simulink library "NCS_Library"  (R2019a)
settings: Solver=VariableStepAuto  StartTime=0.0  StopTime=10.0  RelTol=1e-3
values from neighbouring files (symbols this model uses):
  A = 10    [Parameter.m]
  band = 100000000    [Parameter.m]
  BER = 0    [Parameter.m]
  c = 5000000    [Parameter.m]
  c1 = 4.33    [Parameter.m]
  c2 = 3.16    [Parameter.m]
  CAN2EthernetDelay = 0.000    (= 0)    [Parameter.m]
  cR = 1.5*10^-3    (= 0.0015)    [Parameter.m]
  cw = (cwE * 2 + cwM * (nW_ges-2))/nW_ges    (= 0.1475)    [Parameter.m]
  cwE = 0.35    [Parameter.m]
  cwM = 0.08    [Parameter.m]
  Cycle_Controller = 0    [Parameter.m]
  CyclePLC = 24/1000    (= 0.024)    [Parameter.m]
  d = 800000    [Parameter.m]
  Dr = 0.92    [Parameter.m]
  Ethernet2CANDelay = 0.005    [Parameter.m]
  F_konst = 70892    [Parameter.m]
  FA = 100000    [Parameter.m]
  FB_WB_max = 10000    [Parameter.m]
  FBel_an = iG*nG*F_KZmax*nBan*R_mR/(Dr/2)    (= 28197.4297239)    [Parameter.m]
  FBel_frei = iG*nG*F_KZmax*nBfrei*R_mW/(Dr/2)    (= 29270.6882948)    [Parameter.m]
  Fmaxdyn = 300000    [Parameter.m]
  g = 9.81    [Parameter.m]
  i = 0    [Parameter.m]
  J = 1/2*mA*(Dr/2)^2    (= 158.7)    [Parameter.m]
  k1 = 0.095    [Parameter.m]
  k2 = 9.26/3.6    (= 2.57222222222)    [Parameter.m]
  k3 = 4.63/3.6    (= 1.28611111111)    [Parameter.m]
  mges = 58000    [Parameter.m]
  mu = [mu1 mu2]    [Parameter.m]
  muBel1 = 0.42    [Parameter.m]
  muBel2 = 0.36    [Parameter.m]
  n = 0.001    [Parameter.m]
  n_Mg = 4    [Parameter.m]
  n_WB = 4    [Parameter.m]
  nA = 4    [Parameter.m]
  nBan = 2    [Parameter.m]
  nBfrei = 3    [Parameter.m]
  nM = 4    [Parameter.m]
  nW_an = 4    [Parameter.m]
  P_max = 8200000    [Parameter.m]
  Q = 10    [Parameter.m]
  r_reib = 600    [Parameter.m]
  rho = 1.08    [Parameter.m]
  rhoL = 1.225    [Parameter.m]
  Size = 8    [Parameter.m]
  slip = [s1 s2]    [Parameter.m]
  tol = 0.05    [Parameter.m]
  v00 = 100/3.6    (= 27.7777777778)    [Parameter.m]
  v_grenz = 60/3.6    (= 16.6666666667)    [Parameter.m]
  v_opt = 75/3.6    (= 20.8333333333)    [Parameter.m]
  W_opt = 0.5    [Parameter.m]
  WB = 1    [Parameter.m]
  y_opt = sqrt(W_opt)/((1+sqrt(W_opt))^2+W_opt)    [Parameter.m]
undefined symbols (not defined in the file or in its folder): BUSCapacity, CableLength, controlGate, D_dyn, D_mg, EnableBurst, EnableToF, entity, Entity_out, Gate, Gate_4, Gate_5, Gate_ACK, Gate_copy, Gate_RX, getData, gettime, I_dyn, I_mg, m, magnitude, P_dyn, P_mg, ReadAttributes, readdata, ReadData, ReadSize, sigbuilder_block, Timeout, ToB, ToF, v0, v_d, v_soll
libraries: simulink x176, $bdroot x102
(part 5 of 12)

== system NCS_Library/Controller/Cookie/Braking Controller/konstante Fahrt ==
  v : Inport
  Add : Sum  Inputs=|+-
  Constant : Constant  Value=v_d
  Display : Display
  Display1 : Display
  Gain : Gain  Gain=-1
  Mux2 : Mux  Inputs=3
  PID Controller : simulink/Continuous/PID Controller  Controller=PID  Form=Parallel  TimeDomain=Continuous-time  SampleTime=-1  IntegratorMethod=Forward Euler  FilterMethod=Forward Euler  ControllerParametersSource=internal  P=0.05  I=0.025  D=0.001  UseFilter=on  N=100  TunerSelectOption=Transfer Function Based (PID Tuner App)  InitialConditionSource=internal  InitialConditionForIntegrator=0  InitialConditionForFilter=0  DifferentiatorICPrevScaledInput=0  ExternalReset=none  TrackingMode=off  Kt=1  LimitOutput=off  UpperSaturationLimit=inf  LowerSaturationLimit=-inf  LinearizeAsGain=on  AntiWindupMode=none  Kb=1  POutMin=[]  POutMax=[]  IOutMin=[]  IOutMax=[]  DOutMin=[]  DOutMax=[]  NOutMin=[]  NOutMax=[]  SumOutMin=[]  SumOutMax=[]  SaturationOutMin=[]  SaturationOutMax=[]  PParamMin=[]  PParamMax=[]  IParamMin=[]  IParamMax=[]  DParamMin=[]  DParamMax=[]  NParamMin=[]  NParamMax=[]  KbParamMin=[]  KbParamMax=[]  KtParamMin=[]  KtParamMax=[]  KbOutMin=[]  KbOutMax=[]  KtOutMin=[]  KtOutMax=[]  IntegratorOutMin=[]  IntegratorOutMax=[]  FilterOutMin=[]  FilterOutMax=[]  SumI1OutMin=[]  SumI1OutMax=[]  SumI2OutMin=[]  SumI2OutMax=[]  SumI3OutMin=[]  SumI3OutMax=[]  SumI4OutMin=[]  SumI4OutMax=[]  SumDOutMin=[]  SumDOutMax=[]  DifferentiatorOutMin=[]  DifferentiatorOutMax=[]  FilterDiffOutCoefMin=[]  FilterDiffOutCoefMax=[]  ReciprocalOutMin=[]  ReciprocalOutMax=[]  SumDenOutMin=[]  SumDenOutMax=[]  SumNumOutMin=[]  SumNumOutMax=[]  DivideOutMin=[]  DivideOutMax=[]  IntegratorContinuousStateAttributes=''  IntegratorStateMustResolveToSignalObject=off  IntegratorRTWStateStorageClass=Auto  FilterContinuousStateAttributes=''  FilterStateMustResolveToSignalObject=off  FilterRTWStateStorageClass=Auto  ParallelPVariant=InternalParameters  IdealPVariant=Disabled  IVariant=InternalParameters  DVariant=InternalParameters  IntegratorVariant=Continuous  SatVariant=Disabled  AWVariant=Passthrough  PCopyVariant=Disabled  TRVariant=Disabled  FdbkBlocksVariant=Forward  IdealPFdbkVariant=Disabled  SatFdbkVariant=Disabled  DerivativeFilterVariant=ContFilter  NVariant=InternalParameters  NCopyVariant=Disabled  FilterICVariant=InternalICsFilter  IntegratorICVariant=InternalICs  ExternalResetVariant=Disabled  TRSumVariant=Passthrough  SumFdbkVariant=Disabled  SumVariant=Sum_PID
  PID Controller1 : simulink/Continuous/PID Controller  Controller=PID  Form=Parallel  TimeDomain=Continuous-time  SampleTime=-1  IntegratorMethod=Forward Euler  FilterMethod=Forward Euler  ControllerParametersSource=internal  P=10  I=100  D=0  UseFilter=on  N=100  TunerSelectOption=Transfer Function Based (PID Tuner App)  InitialConditionSource=internal  InitialConditionForIntegrator=0  InitialConditionForFilter=0  DifferentiatorICPrevScaledInput=0  ExternalReset=none  TrackingMode=off  Kt=1  LimitOutput=off  UpperSaturationLimit=inf  LowerSaturationLimit=-inf  LinearizeAsGain=on  AntiWindupMode=none  Kb=1  POutMin=[]  POutMax=[]  IOutMin=[]  IOutMax=[]  DOutMin=[]  DOutMax=[]  NOutMin=[]  NOutMax=[]  SumOutMin=[]  SumOutMax=[]  SaturationOutMin=[]  SaturationOutMax=[]  PParamMin=[]  PParamMax=[]  IParamMin=[]  IParamMax=[]  DParamMin=[]  DParamMax=[]  NParamMin=[]  NParamMax=[]  KbParamMin=[]  KbParamMax=[]  KtParamMin=[]  KtParamMax=[]  KbOutMin=[]  KbOutMax=[]  KtOutMin=[]  KtOutMax=[]  IntegratorOutMin=[]  IntegratorOutMax=[]  FilterOutMin=[]  FilterOutMax=[]  SumI1OutMin=[]  SumI1OutMax=[]  SumI2OutMin=[]  SumI2OutMax=[]  SumI3OutMin=[]  SumI3OutMax=[]  SumI4OutMin=[]  SumI4OutMax=[]  SumDOutMin=[]  SumDOutMax=[]  DifferentiatorOutMin=[]  DifferentiatorOutMax=[]  FilterDiffOutCoefMin=[]  FilterDiffOutCoefMax=[]  ReciprocalOutMin=[]  ReciprocalOutMax=[]  SumDenOutMin=[]  SumDenOutMax=[]  SumNumOutMin=[]  SumNumOutMax=[]  DivideOutMin=[]  DivideOutMax=[]  IntegratorContinuousStateAttributes=''  IntegratorStateMustResolveToSignalObject=off  IntegratorRTWStateStorageClass=Auto  FilterContinuousStateAttributes=''  FilterStateMustResolveToSignalObject=off  FilterRTWStateStorageClass=Auto  ParallelPVariant=InternalParameters  IdealPVariant=Disabled  IVariant=InternalParameters  DVariant=InternalParameters  IntegratorVariant=Continuous  SatVariant=Disabled  AWVariant=Passthrough  PCopyVariant=Disabled  TRVariant=Disabled  FdbkBlocksVariant=Forward  IdealPFdbkVariant=Disabled  SatFdbkVariant=Disabled  DerivativeFilterVariant=ContFilter  NVariant=InternalParameters  NCopyVariant=Disabled  FilterICVariant=InternalICsFilter  IntegratorICVariant=InternalICs  ExternalResetVariant=Disabled  TRSumVariant=Passthrough  SumFdbkVariant=Disabled  SumVariant=Sum_PID
  Saturation : Saturate  UpperLimit=1  LowerLimit=-1  ZeroCross=off
  Saturation1 : Saturate  UpperLimit=0.01  LowerLimit=0  ZeroCross=off
  fSt1 : Constant  Value=0
  fSt : Outport
  wires:
  Gain/1 -> Saturation/1, Display1/1
  Add/1 -> PID Controller/1, PID Controller1/1, Display/1  "e"
  v/1 -> Add/2  "y_m"
  Constant/1 -> Add/1  "w"
  fSt1/1 -> Mux2/2  "f_St,pneumatic"
  Mux2/1 -> fSt/1
  PID Controller/1 -> Gain/1  "u"
  PID Controller1/1 -> Saturation1/1  "u"
  Saturation/1 -> Mux2/1  "f_St,dyn"
  Saturation1/1 -> Mux2/3  "f_St,mg"

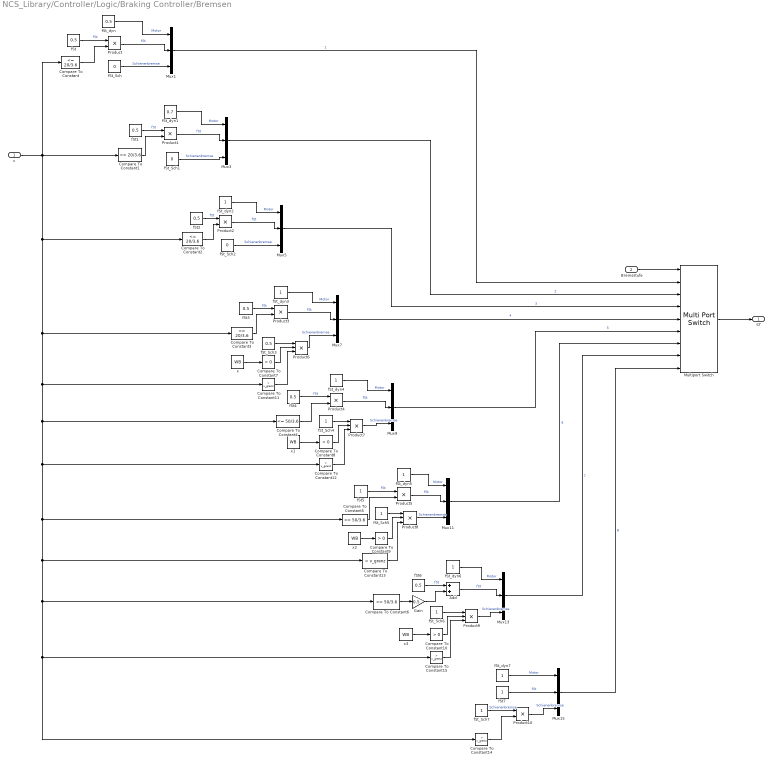
== system NCS_Library/Controller/Logic/Braking Controller/Bremsen ==
  v : Inport
  Bremsstufe : Inport  Port=2
  Add : Sum
  Compare To Constant{,1..3} (4 alike) : simulink/Logic and Bit Operations/Compare To Constant  relop=<=  const=20/3.6  OutDataTypeStr=boolean
  Compare To Constant{7..10} (4 alike) : simulink/Logic and Bit Operations/Compare To Constant  relop=>  const=0  OutDataTypeStr=boolean
  Compare To Constant{11..15} (5 alike) : simulink/Logic and Bit Operations/Compare To Constant  relop=>  const=v_grenz  OutDataTypeStr=boolean
  Compare To Constant4 : simulink/Logic and Bit Operations/Compare To Constant  relop=<=  const=50/3.6  OutDataTypeStr=boolean
  Compare To Constant5 : simulink/Logic and Bit Operations/Compare To Constant  relop=<=  const=50/3.6  OutDataTypeStr=boolean
  Compare To Constant6 : simulink/Logic and Bit Operations/Compare To Constant  relop=<=  const=50/3.6  OutDataTypeStr=boolean
  Gain : Gain  Gain=0.5
  Multiport Switch : MultiPortSwitch  Inputs=8
  Mux{1,3,5,7,9,11,13,15} (8 alike) : Mux  Inputs=3
  Product{,1..5,10} (7 alike) : Product
  Product{6..9} (4 alike) : Product  Inputs=3
  fSt{,1..4,6} (6 alike) : Constant  Value=0.5
  fSt5 : Constant
  fSt7 : Constant
  fSt_Sch : Constant  Value=0
  fSt_Sch1 : Constant  Value=0
  fSt_Sch2 : Constant  Value=0
  fSt_Sch3 : Constant  Value=0.5
  fSt_Sch{4..7} (4 alike) : Constant
  fSt_dyn : Constant  Value=0.5
  fSt_dyn1 : Constant  Value=0.7
  fSt_dyn{2..7} (6 alike) : Constant
  x{,1..3} (4 alike) : Constant  Value=WB
  ST : Outport
  wires:
  Compare To Constant15/1 -> Product9/3
  Compare To Constant14/1 -> Product10/2
  Product10/1 -> Mux15/3  "Schienenbremse"
  Compare To Constant13/1 -> Product8/3
  Compare To Constant12/1 -> Product7/3
  Compare To Constant11/1 -> Product6/3
  Compare To Constant10/1 -> Product9/2
  x3/1 -> Compare To Constant10/1
  fSt_Sch6/1 -> Product9/1
  Compare To Constant9/1 -> Product8/2
  x2/1 -> Compare To Constant9/1
  fSt_Sch5/1 -> Product8/1
  Compare To Constant8/1 -> Product7/2
  x1/1 -> Compare To Constant8/1
  fSt_Sch4/1 -> Product7/1
  Compare To Constant7/1 -> Product6/2
  x/1 -> Compare To Constant7/1
  fSt_Sch3/1 -> Product6/1
  Gain/1 -> Add/2
  fSt6/1 -> Add/1  "fSt"
  Compare To Constant6/1 -> Gain/1
  fSt5/1 -> Product5/1  "fSt"
  Compare To Constant5/1 -> Product5/2
  fSt4/1 -> Product4/1  "fSt"
  Compare To Constant4/1 -> Product4/2
  fSt3/1 -> Product3/1  "fSt"
  Compare To Constant3/1 -> Product3/2
  fSt2/1 -> Product2/1  "fSt"
  Compare To Constant2/1 -> Product2/2
  Compare To Constant1/1 -> Product1/2
  fSt1/1 -> Product1/1  "fSt"
  v/1 -> Compare To Constant1/1, Compare To Constant/1, Compare To Constant2/1, Compare To Constant3/1, Compare To Constant11/1, Compare To Constant4/1, Compare To Constant12/1, Compare To Constant5/1, Compare To Constant14/1, Compare To Constant15/1, Compare To Constant6/1, Compare To Constant13/1
  Compare To Constant/1 -> Product/2
  fSt/1 -> Product/1  "fSt"
  Bremsstufe/1 -> Multiport Switch/1
  Mux15/1 -> Multiport Switch/9  "8"
  fSt_dyn7/1 -> Mux15/1  "Motor"
  fSt_Sch7/1 -> Product10/1  "Schienenbremse"
  fSt7/1 -> Mux15/2  "fSt"
  Mux13/1 -> Multiport Switch/8  "7"
  fSt_dyn6/1 -> Mux13/1  "Motor"
  Product9/1 -> Mux13/3  "Schienenbremse"
  Add/1 -> Mux13/2  "fSt"
  Mux11/1 -> Multiport Switch/7  "6"
  fSt_dyn5/1 -> Mux11/1  "Motor"
  Product8/1 -> Mux11/3  "Schienenbremse"
  Product5/1 -> Mux11/2  "fSt"
  Mux9/1 -> Multiport Switch/6  "5"
  fSt_dyn4/1 -> Mux9/1  "Motor"
  Product7/1 -> Mux9/3  "Schienenbremse"
  Product4/1 -> Mux9/2  "fSt"
  Mux7/1 -> Multiport Switch/5  "4"
  fSt_dyn3/1 -> Mux7/1  "Motor"
  Product6/1 -> Mux7/3  "Schienenbremse"
  Product3/1 -> Mux7/2  "fSt"
  Mux5/1 -> Multiport Switch/4  "3"
  fSt_dyn2/1 -> Mux5/1  "Motor"
  fSt_Sch2/1 -> Mux5/3  "Schienenbremse"
  Product2/1 -> Mux5/2  "fSt"
  Mux3/1 -> Multiport Switch/3  "2"
  fSt_dyn1/1 -> Mux3/1  "Motor"
  fSt_Sch1/1 -> Mux3/3  "Schienenbremse"
  Product1/1 -> Mux3/2  "fSt"
  Mux1/1 -> Multiport Switch/2  "1"
  fSt_dyn/1 -> Mux1/1  "Motor"
  fSt_Sch/1 -> Mux1/3  "Schienenbremse"
  Product/1 -> Mux1/2  "fSt"
  Multiport Switch/1 -> ST/1

== system NCS_Library/Controller/Logic/Braking Controller/Leerlauf ==
  F_B : Constant  Value=0
  Mux1 : Mux  Inputs=3
  fSt : Constant  Value=0
  fSt_Sch : Constant  Value=0
  ST : Outport
  wires:
  Mux1/1 -> ST/1
  fSt_Sch/1 -> Mux1/3  "Schienenbremse"
  fSt/1 -> Mux1/2  "fSt"
  F_B/1 -> Mux1/1  "Motor"

== system NCS_Library/Controller/Logic/Braking Controller/Notbremsung ==
  v : Inport
  Compare To Constant : simulink/Logic and Bit Operations/Compare To Constant  relop=>  const=v_grenz  OutDataTypeStr=boolean
  Mux2 : Mux  Inputs=3
  Product9 : Product
  fSt : Constant
  fSt_Sch : Constant
  fSt_dyn : Constant
  ST : Outport
  wires:
  Compare To Constant/1 -> Product9/2
  v/1 -> Compare To Constant/1
  fSt_Sch/1 -> Product9/1  "Schienenbremse"
  fSt_dyn/1 -> Mux2/1  "fSt_dyn"
  Product9/1 -> Mux2/3  "Schienenbremse"
  fSt/1 -> Mux2/2  "fSt"
  Mux2/1 -> ST/1

== system NCS_Library/Controller/Logic/Braking Controller/konstante Fahrt ==
  v : Inport
  Display{,1..3} (4 alike) : Display
  Fahrwiderstand : Subsystem
  Mux2 : Mux  Inputs=3
  Saturation : Saturate  UpperLimit=1  LowerLimit=0  ZeroCross=off
  Saturation1 : Saturate  UpperLimit=1  LowerLimit=0  ZeroCross=off
  Subsystem : Subsystem
  Subsystem1 : Subsystem
  WB Bremse pro Wagen : Subsystem
  fSt1 : Constant  Value=0
  verfügbare Dynamische Bremskraft : Subsystem
  fSt : Outport
  wires:
  verfügbare Dynamische Bremskraft/1(F_B,dyn_max) -> Subsystem1/2(F_B,dyn_max), Subsystem/2(FB)
  Fahrwiderstand/1(F_W) -> Subsystem1/1(F_W), Subsystem/1(FW)  "FW"
  fSt1/1 -> Mux2/2  "fSt"
  Mux2/1 -> fSt/1
  v/1 -> Subsystem1/4(v), WB Bremse pro Wagen/1(v), Fahrwiderstand/1(v), verfügbare Dynamische Bremskraft/1(v)
  Subsystem/1(Motor) -> Display/1, Saturation/1
  WB Bremse pro Wagen/1(F_B,WB) -> Subsystem1/3(F_B,WB)  "F_B,WB"
  Subsystem1/1(Schienenbremse) -> Display2/1, Saturation1/1
  Saturation/1 -> Display1/1, Mux2/1
  Saturation1/1 -> Display3/1, Mux2/3

== system NCS_Library/Controller/Logic/Subsystem/Triggered Subsystem ==
  In1 : Inport
  Trigger : TriggerPort  VariantControl=Variant
  Out1 : Outport
  wires:
  In1/1 -> Out1/1

== system NCS_Library/Controller/Logic/Subsystem/Triggered Subsystem1 ==
  In1 : Inport
  Trigger : TriggerPort  TriggerType=falling  VariantControl=Variant
  Out1 : Outport
  wires:
  In1/1 -> Out1/1

== system NCS_Library/Controller/Logic/Subsystem1/Triggered Subsystem ==
  In1 : Inport
  Trigger : TriggerPort  VariantControl=Variant
  Out1 : Outport
  wires:
  In1/1 -> Out1/1

== system NCS_Library/Controller/Logic/Subsystem1/Triggered Subsystem1 ==
  In1 : Inport
  Trigger : TriggerPort  TriggerType=falling  VariantControl=Variant
  Out1 : Outport
  wires:
  In1/1 -> Out1/1

== system NCS_Library/Network/Applications/Failure Control/Simulink Function ==
  f : TriggerPort  TriggerType=function-call  IsSimulinkFunction=on  FunctionName=DeleteData  FunctionVisibility=scoped  VariantControl=(inherit)
  Constant : Constant  Value=zeros(3,20)
  y : ArgOut  DisableCoverage=on  PortDimensions=[3 20]  ArgumentName=Data
  wires:
  Constant/1 -> y/1

== system NCS_Library/Network/Applications/Watch Dog/Timeout Watch Dog/GetTime ==
  f : TriggerPort  TriggerType=function-call  VariantControl=(inherit)
      settings: CopyFcn=Stateflow.SLINSF.SimulinkMan.removeBlockPreDeleteFcn  PreDeleteFcn=Stateflow.SLINSF.SimulinkMan.unsafePredeleteFcn
  Digital Clock : DigitalClock  SampleTime=-1
  Time : Outport
  wires:
  Digital Clock/1 -> Time/1

== system NCS_Library/Network/CAN/CAN BUS/Simulink Function ==
  setLossState : TriggerPort  TriggerType=function-call  IsSimulinkFunction=on  FunctionName=setLossState  FunctionVisibility=scoped  VariantControl=Variant
  Constant : Constant
  Constant1 : Constant  Value=0
  Switch : Switch  Criteria=u2 > Threshold  Threshold=LossRate  ZeroCross=off
  Uniform Random Number : UniformRandomNumber  Minimum=0  Seed=724572
  state : ArgOut  ArgumentName=state
  wires:
  Uniform Random Number/1 -> Switch/2
  Constant/1 -> Switch/3
  Constant1/1 -> Switch/1
  Switch/1 -> state/1

== system NCS_Library/Network/CAN/CAN BUS/Simulink Function1 ==
  controlGate : TriggerPort  TriggerType=function-call  IsSimulinkFunction=on  FunctionName=controlGate  FunctionVisibility=scoped  VariantControl=Variant
  Message Send : MessageSend  OutputPortMessageModes=m
      settings: InputPortMap=u1
  u : ArgIn  DisableCoverage=on  ArgumentName=u
  ctrl : Outport
  wires:
  Message Send/1 -> ctrl/1
  u/1 -> Message Send/1

== system NCS_Library/Network/CAN/CAN BUS1/Simulink Function ==
  setLossState : TriggerPort  TriggerType=function-call  IsSimulinkFunction=on  FunctionName=setLossState  FunctionVisibility=scoped  VariantControl=Variant
  Constant : Constant
  Constant1 : Constant  Value=0
  Switch : Switch  Criteria=u2 > Threshold  Threshold=LossRate  ZeroCross=off
  Uniform Random Number : UniformRandomNumber  Minimum=0  Seed=724572
  state : ArgOut  ArgumentName=state
  wires:
  Switch/1 -> state/1
  Constant1/1 -> Switch/1
  Constant/1 -> Switch/3
  Uniform Random Number/1 -> Switch/2

== system NCS_Library/Network/CAN/CAN BUS1/Simulink Function1 ==
  controlGate : TriggerPort  TriggerType=function-call  IsSimulinkFunction=on  FunctionName=controlGate  FunctionVisibility=scoped  VariantControl=Variant
  Message Send : MessageSend  OutputPortMessageModes=m
      settings: InputPortMap=u1
  u : ArgIn  DisableCoverage=on  ArgumentName=u
  ctrl : Outport
  wires:
  u/1 -> Message Send/1
  Message Send/1 -> ctrl/1

== system NCS_Library/Network/CAN/CAN Node 1/Re-Transmission Control ==
  IN : Inport
  ReTX : Inport  Port=2
  Reset : Inport  Port=3
  Discard Saved Message upon Success : EntityGate  InputPortMessageModes=m,m  OutputPortMessageModes=m  OperatingMode=Release gate
  Entity Sink : EntityTerminator  InputPortMessageModes=m  NumberEntitiesArrived=on
      settings: OutputPortMap=o0
  Re-Transmission Decision : EntityOutputSwitch  InputPortMessageModes=m  OutputPortMessageModes=m,m  SwitchAttributeName=Attribute1
  Re-transmit Saved Message upon Failure : EntityGate  InputPortMessageModes=m,m  OutputPortMessageModes=m  OperatingMode=Release gate
  OUT : Outport
  #TX : Outport  Port=2
  wires:
  IN/1 -> Re-Transmission Decision/1
  Re-Transmission Decision/1 -> Re-transmit Saved Message upon Failure/2
  Re-transmit Saved Message upon Failure/1 -> OUT/1
  Re-Transmission Decision/2 -> Discard Saved Message upon Success/2
  Discard Saved Message upon Success/1 -> Entity Sink/1
  Entity Sink/1 -> #TX/1
  ReTX/1 -> Re-transmit Saved Message upon Failure/1
  Reset/1 -> Discard Saved Message upon Success/1

== system NCS_Library/Network/CAN/CAN Node 1/Reception Control/Compute ==
  rx_id : Inport  OutDataTypeStr=double  PortDimensions=1
  loss : Inport  Port=2  OutDataTypeStr=double  PortDimensions=1
  rx_rtr : Inport  Port=3  OutDataTypeStr=double  PortDimensions=1
  rx_data : Inport  Port=4  OutDataTypeStr=double  PortDimensions=1
  tx_id : Inport  Port=5  OutDataTypeStr=double  PortDimensions=1
  tx_rtr : Inport  Port=6  OutDataTypeStr=double  PortDimensions=1
  tx_data : Inport  Port=7  OutDataTypeStr=double  PortDimensions=1
  f : TriggerPort  TriggerType=function-call  VariantControl=Variant
      settings: CopyFcn=Stateflow.SLINSF.SimulinkMan.removeBlockPreDeleteFcn  PreDeleteFcn=Stateflow.SLINSF.SimulinkMan.unsafePredeleteFcn
  Lookup Table : Lookup  InputValues=IDRange  Table=2*ones(1,length(IDRange))-IDSubscription  LUTDesignUseExistingBP=off  LUTDesignAbsError=NaN
  MATLAB Function : MATLAB Function  TreatAsAtomicUnit=on
  Sum : Sum  Inputs=|++
  Status : Outport
  Ack : Outport  Port=2
  wires:
  MATLAB Function/1(ACK) -> Ack/1
  Sum/1 -> Status/1
  tx_rtr/1 -> MATLAB Function/5(RTR1)
  tx_data/1 -> MATLAB Function/6(Data1)
  rx_data/1 -> MATLAB Function/3(Data0)
  loss/1 -> MATLAB Function/7(Loss), Sum/2
  Lookup Table/1 -> Sum/1
  rx_id/1 -> Lookup Table/1, MATLAB Function/1(ID0)
  rx_rtr/1 -> MATLAB Function/2(RTR0)
  tx_id/1 -> MATLAB Function/4(ID1)

== system NCS_Library/Network/CAN/CAN Node 1/Signal To CAN Message ==
  Data : Inport
  Entity Generator : EntityGenerator  OutputPortMessageModes=m  Period=T_Tx  GenerateEntityAtSimulationStart=off  GenerateAction=[entity.ID,entity.RTR,entity.Size,entity.Data,entity.CommDelay,entity.Time, entity.SensorType] = initMessage();  AttributeName=ID|RTR|Size|Data|CommDelay|RndLoss  AttributeInitialValue=1|1|1|1|1|0  EntityType=Bus object  EntityTypeName=CAN_Message  EntityPriority=MsgID
  Set the Attributes of Messages : Subsystem  TreatAsAtomicUnit=on
  MsgOut : Outport
  wires:
  Data/1 -> Set the Attributes of Messages/1(InData)
  Entity Generator/1 -> MsgOut/1

== system NCS_Library/Network/CAN/CAN Node 1/Simulink Function ==
  controlGate : TriggerPort  TriggerType=function-call  IsSimulinkFunction=on  FunctionName=controlGate  FunctionVisibility=scoped  VariantControl=Variant
  Message Send : MessageSend  OutputPortMessageModes=m
      settings: InputPortMap=u1
  u : ArgIn  DisableCoverage=on  ArgumentName=u
  ctrl : Outport
  wires:
  Message Send/1 -> ctrl/1
  u/1 -> Message Send/1

== system NCS_Library/Network/CAN/CAN Node 1/Simulink Function1 ==
  getData : TriggerPort  TriggerType=function-call  IsSimulinkFunction=on  FunctionName=getData  FunctionVisibility=scoped  VariantControl=Variant
  Mux : Mux  Inputs=3
  u : ArgIn  DisableCoverage=on  ArgumentName=u
  u1 : ArgIn  DisableCoverage=on  Port=2  PortDimensions=[3 1]  ArgumentName=f_St
  data : Outport
  f_St : Outport  Port=2
  wires:
  u/1 -> Mux/1, Mux/3, Mux/2
  u1/1 -> f_St/1
  Mux/1 -> data/1

== system NCS_Library/Network/CAN/CAN Node 2/Re-Transmission Control ==
  IN : Inport
  ReTX : Inport  Port=2
  Reset : Inport  Port=3
  Discard Saved Message upon Success : EntityGate  InputPortMessageModes=m,m  OutputPortMessageModes=m  OperatingMode=Release gate
  Entity Sink : EntityTerminator  InputPortMessageModes=m  NumberEntitiesArrived=on
      settings: OutputPortMap=o0
  Re-Transmission Decision : EntityOutputSwitch  InputPortMessageModes=m  OutputPortMessageModes=m,m  SwitchAttributeName=Attribute1
  Re-transmit Saved Message upon Failure : EntityGate  InputPortMessageModes=m,m  OutputPortMessageModes=m  OperatingMode=Release gate
  OUT : Outport
  #TX : Outport  Port=2
  wires:
  Reset/1 -> Discard Saved Message upon Success/1
  ReTX/1 -> Re-transmit Saved Message upon Failure/1
  Entity Sink/1 -> #TX/1
  Discard Saved Message upon Success/1 -> Entity Sink/1
  Re-Transmission Decision/2 -> Discard Saved Message upon Success/2
  Re-transmit Saved Message upon Failure/1 -> OUT/1
  Re-Transmission Decision/1 -> Re-transmit Saved Message upon Failure/2
  IN/1 -> Re-Transmission Decision/1

== system NCS_Library/Network/CAN/CAN Node 2/Reception Control/Compute ==
  rx_id : Inport  OutDataTypeStr=double  PortDimensions=1
  loss : Inport  Port=2  OutDataTypeStr=double  PortDimensions=1
  rx_rtr : Inport  Port=3  OutDataTypeStr=double  PortDimensions=1
  rx_data : Inport  Port=4  OutDataTypeStr=double  PortDimensions=1
  tx_id : Inport  Port=5  OutDataTypeStr=double  PortDimensions=1
  tx_rtr : Inport  Port=6  OutDataTypeStr=double  PortDimensions=1
  tx_data : Inport  Port=7  OutDataTypeStr=double  PortDimensions=1
  f : TriggerPort  TriggerType=function-call  VariantControl=Variant
      settings: CopyFcn=Stateflow.SLINSF.SimulinkMan.removeBlockPreDeleteFcn  PreDeleteFcn=Stateflow.SLINSF.SimulinkMan.unsafePredeleteFcn
  Lookup Table : Lookup  InputValues=IDRange  Table=2*ones(1,length(IDRange))-IDSubscription  LUTDesignUseExistingBP=off  LUTDesignAbsError=NaN
  MATLAB Function : MATLAB Function  TreatAsAtomicUnit=on
  Sum : Sum  Inputs=|++
  Status : Outport
  Ack : Outport  Port=2
  wires:
  tx_id/1 -> MATLAB Function/4(ID1)
  rx_rtr/1 -> MATLAB Function/2(RTR0)
  rx_id/1 -> MATLAB Function/1(ID0), Lookup Table/1
  Lookup Table/1 -> Sum/1
  loss/1 -> Sum/2, MATLAB Function/7(Loss)
  rx_data/1 -> MATLAB Function/3(Data0)
  tx_data/1 -> MATLAB Function/6(Data1)
  tx_rtr/1 -> MATLAB Function/5(RTR1)
  Sum/1 -> Status/1
  MATLAB Function/1(ACK) -> Ack/1

== system NCS_Library/Network/CAN/CAN Node 2/Signal To CAN Message ==
  Data : Inport
  Entity Generator : EntityGenerator  OutputPortMessageModes=m  Period=T_Tx  GenerateEntityAtSimulationStart=off  GenerateAction=[entity.ID,entity.RTR,entity.Size,entity.Data,entity.CommDelay,entity.Time, entity.SensorType] = initMessage();  AttributeName=ID|RTR|Size|Data|CommDelay|RndLoss  AttributeInitialValue=1|1|1|1|1|0  EntityType=Bus object  EntityTypeName=CAN_Message  EntityPriority=MsgID
  Set the Attributes of Messages : Subsystem  TreatAsAtomicUnit=on
  MsgOut : Outport
  wires:
  Entity Generator/1 -> MsgOut/1
  Data/1 -> Set the Attributes of Messages/1(InData)

== system NCS_Library/Network/CAN/CAN Node 2/Simulink Function ==
  controlGate : TriggerPort  TriggerType=function-call  IsSimulinkFunction=on  FunctionName=controlGate  FunctionVisibility=scoped  VariantControl=Variant
  Message Send : MessageSend  OutputPortMessageModes=m
      settings: InputPortMap=u1
  u : ArgIn  DisableCoverage=on  ArgumentName=u
  ctrl : Outport
  wires:
  u/1 -> Message Send/1
  Message Send/1 -> ctrl/1

== system NCS_Library/Network/CAN/CAN Node 2/Simulink Function1 ==
  getData : TriggerPort  TriggerType=function-call  IsSimulinkFunction=on  FunctionName=getData  FunctionVisibility=scoped  VariantControl=Variant
  Mux : Mux  Inputs=3
  u : ArgIn  DisableCoverage=on  ArgumentName=u
  u1 : ArgIn  DisableCoverage=on  Port=2  PortDimensions=[3 1]  ArgumentName=f_St
  data : Outport
  f_St : Outport  Port=2
  wires:
  Mux/1 -> data/1
  u1/1 -> f_St/1
  u/1 -> Mux/2, Mux/3, Mux/1

== system NCS_Library/Network/CAN/CAN Node 3/ACK Takt ==
  In : Inport
  Entity Takt : EntityGenerator  OutputPortMessageModes=m  TimeSource=Signal port  Period=7  AttributeName=entity  EntityTypeName=gate  EntityPriority=10  DataInitialValue=1
      settings: InputPortMap=u1
  Entity Terminator13 : EntityTerminator  InputPortMessageModes=m
  Gate ACK : EntityGate  InputPortMessageModes=m,m  OutputPortMessageModes=m
  Offset [s] : Constant  Value=Offset
  Server ACK : EntityServer  InputPortMessageModes=m  OutputPortMessageModes=m  Capacity=1  ServiceTimeValue=0  EntryAction=Gate_ACK(ideal);
  Server Offset : EntityServer  InputPortMessageModes=n,m  OutputPortMessageModes=m  Capacity=inf  ServiceTimeSource=Signal port  ServiceTimeValue=5
      settings: InputPortMap=u0,u2
  Server Takt : EntityServer  InputPortMessageModes=m  OutputPortMessageModes=m  Capacity=1  ServiceTimeValue=0.001  ServiceTimeAttributeName=CommDelay  EntryAction=Gate_ACK(1);  ExitAction=Gate_ACK(ideal);  SortingAttributeName=ID
  Simulink Function3 : Subsystem  TreatAsAtomicUnit=on
  Takt [s] : Constant  Value=Takt
  Out : Outport
  wires:
  Offset [s]/1 -> Server Offset/1
  Takt [s]/1 -> Entity Takt/1
  Server Takt/1 -> Entity Terminator13/1
  Server Offset/1 -> Server Takt/1
  Entity Takt/1 -> Server Offset/2
  Simulink Function3/1(ctrl) -> Gate ACK/1
  In/1 -> Gate ACK/2
  Gate ACK/1 -> Server ACK/1
  Server ACK/1 -> Out/1

== system NCS_Library/Network/CAN/CAN Node 3/RX Takt ==
  In : Inport
  Entity Takt : EntityGenerator  OutputPortMessageModes=m  TimeSource=Signal port  Period=7  AttributeName=entity  EntityTypeName=gate  EntityPriority=10  DataInitialValue=1
      settings: InputPortMap=u1
  Entity Terminator13 : EntityTerminator  InputPortMessageModes=m
  Gate RX : EntityGate  InputPortMessageModes=m,m  OutputPortMessageModes=m
  Offset [s] : Constant  Value=Offset
  Server Offset : EntityServer  InputPortMessageModes=n,m  OutputPortMessageModes=m  Capacity=inf  ServiceTimeSource=Signal port  ServiceTimeValue=5
      settings: InputPortMap=u0,u2
  Server RX : EntityServer  InputPortMessageModes=m  OutputPortMessageModes=m  Capacity=1  ServiceTimeValue=0  EntryAction=Gate_RX(ideal);
  Server Takt : EntityServer  InputPortMessageModes=m  OutputPortMessageModes=m  Capacity=1  ServiceTimeValue=0.001  ServiceTimeAttributeName=CommDelay  EntryAction=Gate_RX(1);  ExitAction=Gate_RX(ideal);  SortingAttributeName=ID
  Simulink Function8 : Subsystem  TreatAsAtomicUnit=on
  Takt [s] : Constant  Value=Takt
  Out : Outport
  wires:
  Server RX/1 -> Out/1
  Gate RX/1 -> Server RX/1
  In/1 -> Gate RX/2
  Simulink Function8/1(ctrl) -> Gate RX/1
  Entity Takt/1 -> Server Offset/2
  Server Offset/1 -> Server Takt/1
  Server Takt/1 -> Entity Terminator13/1
  Takt [s]/1 -> Entity Takt/1
  Offset [s]/1 -> Server Offset/1

== system NCS_Library/Network/CAN/CAN Node 3/Re-Transmission Control ==
  Msg_available : Inport
  ReTX : Inport  Port=2
  Reset : Inport  Port=3
  IN : Inport  Port=4
  Discard Saved Message upon Success : EntityGate  InputPortMessageModes=m,m  OutputPortMessageModes=m  OperatingMode=Release gate
  Drop : EntityOutputSwitch  InputPortMessageModes=m  OutputPortMessageModes=m,m  SwitchAttributeName=Attribute1
  Entity Sink : EntityTerminator  InputPortMessageModes=m  NumberEntitiesArrived=on
      settings: OutputPortMap=o0
  Entity Sink1 : EntityTerminator  InputPortMessageModes=m  NumberEntitiesArrived=on
      settings: OutputPortMap=o0
  Gate : EntityGate  InputPortMessageModes=m,m  OutputPortMessageModes=m
  Re-Transmission Decision : EntityOutputSwitch  InputPortMessageModes=m  OutputPortMessageModes=m,m  SwitchAttributeName=Attribute1
  Re-transmit Saved Message upon Failure : EntityGate  InputPortMessageModes=m,m  OutputPortMessageModes=m  OperatingMode=Release gate
  Scope : Scope
  Scope1 : Scope
  Scope2 : Scope
  OUT : Outport
  #TX : Outport  Port=2
  wires:
  Reset/1 -> Discard Saved Message upon Success/1, Scope1/1
  Re-Transmission Decision/2 -> Discard Saved Message upon Success/2
  Re-transmit Saved Message upon Failure/1 -> OUT/1
  Re-Transmission Decision/1 -> Re-transmit Saved Message upon Failure/2
  IN/1 -> Re-Transmission Decision/1
  Discard Saved Message upon Success/1 -> Entity Sink/1
  Entity Sink/1 -> #TX/1
  Drop/2 -> Entity Sink1/1
  Entity Sink1/1 -> Scope/1
  Msg_available/1 -> Gate/1
  ReTX/1 -> Drop/1, Scope2/1
  Drop/1 -> Gate/2
  Gate/1 -> Re-transmit Saved Message upon Failure/1

== system NCS_Library/Network/CAN/CAN Node 3/Reception Control/Acknowledge ==
  ack_id : Inport  OutDataTypeStr=double  PortDimensions=1
  ack_loss : Inport  Port=2  OutDataTypeStr=double  PortDimensions=1
  ack_rtr : Inport  Port=3  OutDataTypeStr=double  PortDimensions=1
  ack_data : Inport  Port=4  OutDataTypeStr=double  PortDimensions=1
  tx_id : Inport  Port=5  OutDataTypeStr=double  PortDimensions=1
  tx_rtr : Inport  Port=6  OutDataTypeStr=double  PortDimensions=1
  tx_data : Inport  Port=7  OutDataTypeStr=double  PortDimensions=1
  f : TriggerPort  TriggerType=function-call  VariantControl=Variant
      settings: CopyFcn=Stateflow.SLINSF.SimulinkMan.removeBlockPreDeleteFcn  PreDeleteFcn=Stateflow.SLINSF.SimulinkMan.unsafePredeleteFcn
  MATLAB Function : MATLAB Function  TreatAsAtomicUnit=on
  Ack : Outport
  wires:
  tx_id/1 -> MATLAB Function/4(ID1)
  tx_data/1 -> MATLAB Function/6(Data1)
  tx_rtr/1 -> MATLAB Function/5(RTR1)
  MATLAB Function/1(ACK) -> Ack/1
  ack_loss/1 -> MATLAB Function/7(Loss)
  ack_id/1 -> MATLAB Function/1(ID0)
  ack_rtr/1 -> MATLAB Function/2(RTR0)
  ack_data/1 -> MATLAB Function/3(Data0)

== system NCS_Library/Network/CAN/CAN Node 3/Reception Control/Receive ==
  rx_id : Inport  OutDataTypeStr=double  PortDimensions=1
  rx_loss : Inport  Port=2  OutDataTypeStr=double  PortDimensions=1
  f : TriggerPort  TriggerType=function-call  VariantControl=Variant
      settings: CopyFcn=Stateflow.SLINSF.SimulinkMan.removeBlockPreDeleteFcn  PreDeleteFcn=Stateflow.SLINSF.SimulinkMan.unsafePredeleteFcn
  Lookup Table : Lookup  InputValues=IDRange  Table=2*ones(1,length(IDRange))-IDSubscription  LUTDesignUseExistingBP=off  LUTDesignAbsError=NaN
  Scope : Scope
  Scope1 : Scope
  Scope2 : Scope
  Sum : Sum  Inputs=|++
  Status : Outport
  wires:
  Lookup Table/1 -> Sum/1
  rx_loss/1 -> Scope1/1, Sum/2
  Sum/1 -> Scope/1, Status/1
  rx_id/1 -> Scope2/1, Lookup Table/1

== system NCS_Library/Network/CAN/CAN Node 3/Simulink Function ==
  Gate_TX : TriggerPort  TriggerType=function-call  IsSimulinkFunction=on  FunctionName=Gate_TX  FunctionVisibility=scoped  VariantControl=Variant
  Message Send : MessageSend  OutputPortMessageModes=m
      settings: InputPortMap=u1
  u : ArgIn  DisableCoverage=on  ArgumentName=u
  ctrl : Outport
  wires:
  u/1 -> Message Send/1
  Message Send/1 -> ctrl/1

== system NCS_Library/Network/CAN/CAN Node 3/Simulink Function1 ==
  getData : TriggerPort  TriggerType=function-call  IsSimulinkFunction=on  FunctionName=getData  FunctionVisibility=scoped  VariantControl=Variant
  u : ArgIn  DisableCoverage=on  ArgumentName=u
  data : Outport
  wires:
  u/1 -> data/1

== system NCS_Library/Network/CAN/CAN Node 3/Simulink Function2 ==
  Msg_available : TriggerPort  TriggerType=function-call  IsSimulinkFunction=on  FunctionName=Msg_available  FunctionVisibility=scoped  VariantControl=Variant
  Message Send : MessageSend  OutputPortMessageModes=m
      settings: InputPortMap=u1
  u : ArgIn  DisableCoverage=on  ArgumentName=u
  ctrl : Outport
  wires:
  Message Send/1 -> ctrl/1
  u/1 -> Message Send/1

== system NCS_Library/Network/CAN/CAN Node 4/ACK Takt ==
  In : Inport
  Entity Takt : EntityGenerator  OutputPortMessageModes=m  TimeSource=Signal port  Period=7  AttributeName=entity  EntityTypeName=gate  EntityPriority=10  DataInitialValue=1
      settings: InputPortMap=u1
  Entity Terminator13 : EntityTerminator  InputPortMessageModes=m
  Gate ACK : EntityGate  InputPortMessageModes=m,m  OutputPortMessageModes=m
  Offset [s] : Constant  Value=Offset
  Server ACK : EntityServer  InputPortMessageModes=m  OutputPortMessageModes=m  Capacity=1  ServiceTimeValue=0  EntryAction=Gate_ACK(ideal);
  Server Offset : EntityServer  InputPortMessageModes=n,m  OutputPortMessageModes=m  Capacity=inf  ServiceTimeSource=Signal port  ServiceTimeValue=5
      settings: InputPortMap=u0,u2
  Server Takt : EntityServer  InputPortMessageModes=m  OutputPortMessageModes=m  Capacity=1  ServiceTimeValue=0.001  ServiceTimeAttributeName=CommDelay  EntryAction=Gate_ACK(1);  ExitAction=Gate_ACK(ideal);  SortingAttributeName=ID
  Simulink Function3 : Subsystem  TreatAsAtomicUnit=on
  Takt [s] : Constant  Value=Takt
  Out : Outport
  wires:
  Server ACK/1 -> Out/1
  Gate ACK/1 -> Server ACK/1
  In/1 -> Gate ACK/2
  Simulink Function3/1(ctrl) -> Gate ACK/1
  Entity Takt/1 -> Server Offset/2
  Server Offset/1 -> Server Takt/1
  Server Takt/1 -> Entity Terminator13/1
  Takt [s]/1 -> Entity Takt/1
  Offset [s]/1 -> Server Offset/1

== system NCS_Library/Network/CAN/CAN Node 4/RX Takt ==
  In : Inport
  Entity Takt : EntityGenerator  OutputPortMessageModes=m  TimeSource=Signal port  Period=7  AttributeName=entity  EntityTypeName=gate  EntityPriority=10  DataInitialValue=1
      settings: InputPortMap=u1
  Entity Terminator13 : EntityTerminator  InputPortMessageModes=m
  Gate RX : EntityGate  InputPortMessageModes=m,m  OutputPortMessageModes=m
  Offset [s] : Constant  Value=Offset
  Server Offset : EntityServer  InputPortMessageModes=n,m  OutputPortMessageModes=m  Capacity=inf  ServiceTimeSource=Signal port  ServiceTimeValue=5
      settings: InputPortMap=u0,u2
  Server RX : EntityServer  InputPortMessageModes=m  OutputPortMessageModes=m  Capacity=1  ServiceTimeValue=0  EntryAction=Gate_RX(ideal);
  Server Takt : EntityServer  InputPortMessageModes=m  OutputPortMessageModes=m  Capacity=1  ServiceTimeValue=0.001  ServiceTimeAttributeName=CommDelay  EntryAction=Gate_RX(1);  ExitAction=Gate_RX(ideal);  SortingAttributeName=ID
  Simulink Function8 : Subsystem  TreatAsAtomicUnit=on
  Takt [s] : Constant  Value=Takt
  Out : Outport
  wires:
  Offset [s]/1 -> Server Offset/1
  Takt [s]/1 -> Entity Takt/1
  Server Takt/1 -> Entity Terminator13/1
  Server Offset/1 -> Server Takt/1
  Entity Takt/1 -> Server Offset/2
  Simulink Function8/1(ctrl) -> Gate RX/1
  In/1 -> Gate RX/2
  Gate RX/1 -> Server RX/1
  Server RX/1 -> Out/1

== system NCS_Library/Network/CAN/CAN Node 4/Re-Transmission Control ==
  Msg_available : Inport
  ReTX : Inport  Port=2
  Reset : Inport  Port=3
  IN : Inport  Port=4
  Discard Saved Message upon Success : EntityGate  InputPortMessageModes=m,m  OutputPortMessageModes=m  OperatingMode=Release gate
  Drop : EntityOutputSwitch  InputPortMessageModes=m  OutputPortMessageModes=m,m  SwitchAttributeName=Attribute1
  Entity Sink : EntityTerminator  InputPortMessageModes=m  NumberEntitiesArrived=on
      settings: OutputPortMap=o0
  Entity Sink1 : EntityTerminator  InputPortMessageModes=m  NumberEntitiesArrived=on
      settings: OutputPortMap=o0
  Gate : EntityGate  InputPortMessageModes=m,m  OutputPortMessageModes=m
  Re-Transmission Decision : EntityOutputSwitch  InputPortMessageModes=m  OutputPortMessageModes=m,m  SwitchAttributeName=Attribute1
  Re-transmit Saved Message upon Failure : EntityGate  InputPortMessageModes=m,m  OutputPortMessageModes=m  OperatingMode=Release gate
  Scope : Scope
  Scope1 : Scope
  Scope2 : Scope
  OUT : Outport
  #TX : Outport  Port=2
  wires:
  Gate/1 -> Re-transmit Saved Message upon Failure/1
  Drop/1 -> Gate/2
  ReTX/1 -> Scope2/1, Drop/1
  Msg_available/1 -> Gate/1
  Entity Sink1/1 -> Scope/1
  Drop/2 -> Entity Sink1/1
  Entity Sink/1 -> #TX/1
  Discard Saved Message upon Success/1 -> Entity Sink/1
  IN/1 -> Re-Transmission Decision/1
  Re-Transmission Decision/1 -> Re-transmit Saved Message upon Failure/2
  Re-transmit Saved Message upon Failure/1 -> OUT/1
  Re-Transmission Decision/2 -> Discard Saved Message upon Success/2
  Reset/1 -> Scope1/1, Discard Saved Message upon Success/1

== system NCS_Library/Network/CAN/CAN Node 4/Reception Control/Acknowledge ==
  ack_id : Inport  OutDataTypeStr=double  PortDimensions=1
  ack_loss : Inport  Port=2  OutDataTypeStr=double  PortDimensions=1
  ack_rtr : Inport  Port=3  OutDataTypeStr=double  PortDimensions=1
  ack_data : Inport  Port=4  OutDataTypeStr=double  PortDimensions=1
  tx_id : Inport  Port=5  OutDataTypeStr=double  PortDimensions=1
  tx_rtr : Inport  Port=6  OutDataTypeStr=double  PortDimensions=1
  tx_data : Inport  Port=7  OutDataTypeStr=double  PortDimensions=1
  f : TriggerPort  TriggerType=function-call  VariantControl=Variant
      settings: CopyFcn=Stateflow.SLINSF.SimulinkMan.removeBlockPreDeleteFcn  PreDeleteFcn=Stateflow.SLINSF.SimulinkMan.unsafePredeleteFcn
  MATLAB Function : MATLAB Function  TreatAsAtomicUnit=on
  Ack : Outport
  wires:
  ack_data/1 -> MATLAB Function/3(Data0)
  ack_rtr/1 -> MATLAB Function/2(RTR0)
  ack_id/1 -> MATLAB Function/1(ID0)
  ack_loss/1 -> MATLAB Function/7(Loss)
  MATLAB Function/1(ACK) -> Ack/1
  tx_rtr/1 -> MATLAB Function/5(RTR1)
  tx_data/1 -> MATLAB Function/6(Data1)
  tx_id/1 -> MATLAB Function/4(ID1)

== system NCS_Library/Network/CAN/CAN Node 4/Reception Control/Receive ==
  rx_id : Inport  OutDataTypeStr=double  PortDimensions=1
  rx_loss : Inport  Port=2  OutDataTypeStr=double  PortDimensions=1
  f : TriggerPort  TriggerType=function-call  VariantControl=Variant
      settings: CopyFcn=Stateflow.SLINSF.SimulinkMan.removeBlockPreDeleteFcn  PreDeleteFcn=Stateflow.SLINSF.SimulinkMan.unsafePredeleteFcn
  Lookup Table : Lookup  InputValues=IDRange  Table=2*ones(1,length(IDRange))-IDSubscription  LUTDesignUseExistingBP=off  LUTDesignAbsError=NaN
  Scope : Scope
  Scope1 : Scope
  Scope2 : Scope
  Sum : Sum  Inputs=|++
  Status : Outport
  wires:
  rx_id/1 -> Lookup Table/1, Scope2/1
  Sum/1 -> Status/1, Scope/1
  rx_loss/1 -> Sum/2, Scope1/1
  Lookup Table/1 -> Sum/1

== system NCS_Library/Network/CAN/CAN Node 4/Simulink Function ==
  Gate_TX : TriggerPort  TriggerType=function-call  IsSimulinkFunction=on  FunctionName=Gate_TX  FunctionVisibility=scoped  VariantControl=Variant
  Message Send : MessageSend  OutputPortMessageModes=m
      settings: InputPortMap=u1
  u : ArgIn  DisableCoverage=on  ArgumentName=u
  ctrl : Outport
  wires:
  Message Send/1 -> ctrl/1
  u/1 -> Message Send/1

== system NCS_Library/Network/CAN/CAN Node 4/Simulink Function1 ==
  getData : TriggerPort  TriggerType=function-call  IsSimulinkFunction=on  FunctionName=getData  FunctionVisibility=scoped  VariantControl=Variant
  u : ArgIn  DisableCoverage=on  ArgumentName=u
  data : Outport
  wires:
  u/1 -> data/1

== system NCS_Library/Network/CAN/CAN Node 4/Simulink Function2 ==
  Msg_available : TriggerPort  TriggerType=function-call  IsSimulinkFunction=on  FunctionName=Msg_available  FunctionVisibility=scoped  VariantControl=Variant
  Message Send : MessageSend  OutputPortMessageModes=m
      settings: InputPortMap=u1
  u : ArgIn  DisableCoverage=on  ArgumentName=u
  ctrl : Outport
  wires:
  u/1 -> Message Send/1
  Message Send/1 -> ctrl/1

== system NCS_Library/Network/CAN/Logik/Fast_to_Slow ==
  note: Process
  note: Downsampling
  In : Inport
  Buffer_Gateway : EntityQueue  InputPortMessageModes=m  OutputPortMessageModes=n,m  Capacity=inf  QueueType=LIFO  NumberEntitiesInBlock=on
      settings: OutputPortMap=o1,o5
  Entity Replicator8 : EntityReplicator  InputPortMessageModes=m  OutputPortMessageModes=m,m
  Entity Replicator9 : EntityReplicator  InputPortMessageModes=m  OutputPortMessageModes=m,m
  Entity Terminator5 : EntityTerminator  InputPortMessageModes=m  NumberEntitiesArrived=on
      settings: OutputPortMap=o0
  Measurement : Subsystem
  Processing Delay : EntityServer  InputPortMessageModes=m  OutputPortMessageModes=m  Capacity=1  ServiceTimeValue=Delay_input  ServiceTimeAttributeName=CommDelay  SortingAttributeName=ID
  Resource Acquirer : EntityResourceAcquirer  InputPortMessageModes=m  OutputPortMessageModes=n,m  ResourceName=Token1  NumberEntitiesInBlock=on
      settings: OutputPortMap=o1,o3
  Resource Releaser : EntityResourceReleaser  InputPortMessageModes=m  OutputPortMessageModes=m  ResourceToRelease=Selected  ResourceName=Token1
  Scope{1..3,13,18} (5 alike) : Scope
  Slow Takt : Subsystem
  Stack : EntityQueue  InputPortMessageModes=m  OutputPortMessageModes=n,m  Capacity=inf  QueueType=LIFO  NumberEntitiesInBlock=on
      settings: OutputPortMap=o1,o5
  Wait Takt : Subsystem
  Out : Outport
  wires:
  Resource Acquirer/1 -> Scope3/1
  Resource Releaser/1 -> Entity Replicator8/1
  Wait Takt/1(Out) -> Resource Acquirer/1
  Resource Acquirer/2 -> Processing Delay/1
  Processing Delay/1 -> Resource Releaser/1
  Slow Takt/1(Out) -> Entity Replicator9/1
  Buffer_Gateway/1 -> Scope13/1
  Entity Replicator9/1 -> Out/1
  In/1 -> Stack/1
  Entity Replicator8/2 -> Entity Terminator5/1
  Stack/1 -> Scope18/1
  Stack/2 -> Wait Takt/1(In)
  Entity Terminator5/1 -> Scope2/1
  Entity Replicator9/2 -> Measurement/1(measure)
  Entity Replicator8/1 -> Buffer_Gateway/1
  Buffer_Gateway/2 -> Slow Takt/1(In)
  Measurement/1(delay) -> Scope1/1

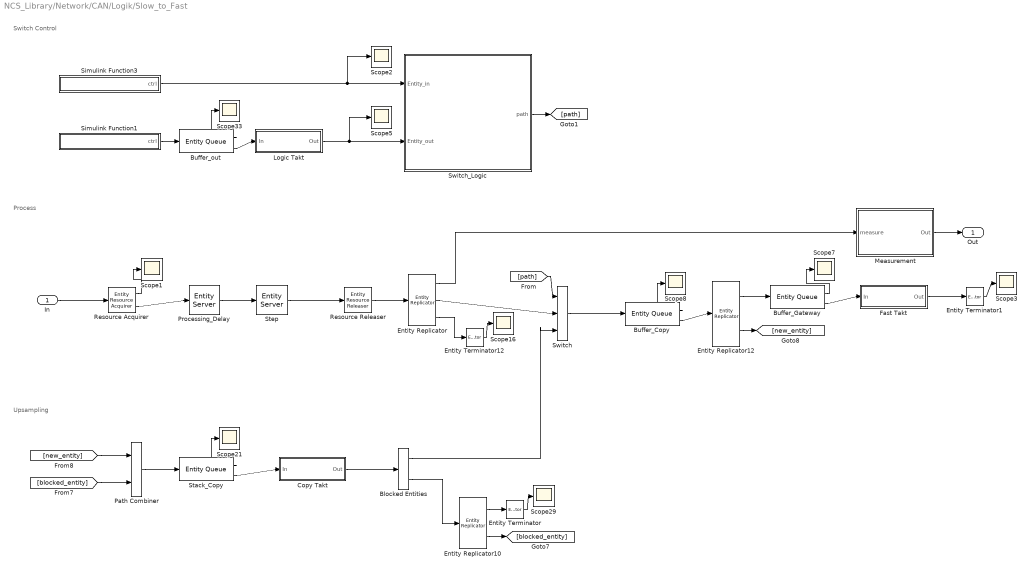
== system NCS_Library/Network/CAN/Logik/Slow_to_Fast ==
  note: Switch Control
  note: Process
  note: Upsampling
  In : Inport
  Blocked Entities : EntityOutputSwitch  InputPortMessageModes=m  OutputPortMessageModes=m,m  SwitchAttributeName=Attribute1
  Buffer_Copy : EntityQueue  InputPortMessageModes=m  OutputPortMessageModes=n,m  Capacity=1000  NumberEntitiesInBlock=on
      settings: OutputPortMap=o1,o5
  Buffer_Gateway : EntityQueue  InputPortMessageModes=m  OutputPortMessageModes=n,m  Capacity=inf  NumberEntitiesInBlock=on
      settings: OutputPortMap=o1,o5
  Buffer_out : EntityQueue  InputPortMessageModes=m  OutputPortMessageModes=n,m  Capacity=inf  NumberEntitiesInBlock=on
      settings: OutputPortMap=o1,o5
  Copy Takt : Subsystem
  Entity Replicator : EntityReplicator  InputPortMessageModes=m  OutputPortMessageModes=m,m,m  NumberReplicas=2
      settings: OutputPortMap=o0,o1,o2
  Entity Replicator10 : EntityReplicator  InputPortMessageModes=m  OutputPortMessageModes=m,m
  Entity Replicator12 : EntityReplicator  InputPortMessageModes=m  OutputPortMessageModes=m,m
  Entity Terminator : EntityTerminator  InputPortMessageModes=m  NumberEntitiesArrived=on
      settings: OutputPortMap=o0
  Entity Terminator1 : EntityTerminator  InputPortMessageModes=m  NumberEntitiesArrived=on
      settings: OutputPortMap=o0
  Entity Terminator12 : EntityTerminator  InputPortMessageModes=m  NumberEntitiesArrived=on
      settings: OutputPortMap=o0
  Fast Takt : Subsystem
  Logic Takt : Subsystem
  Measurement : Subsystem
  Path Combiner : EntityInputSwitch  InputPortMessageModes=m,m  OutputPortMessageModes=m  SwitchingCriterion=From control port
  Processing_Delay : EntityServer  InputPortMessageModes=m  OutputPortMessageModes=m  Capacity=1  ServiceTimeValue=Delay  ServiceTimeAttributeName=CommDelay  EntryAction=%gettime(entity.Time)  SortingAttributeName=ID
  Resource Acquirer : EntityResourceAcquirer  InputPortMessageModes=m  OutputPortMessageModes=n,m  ResourceName=Token1  NumberEntitiesInBlock=on
      settings: OutputPortMap=o1,o3
  Resource Releaser : EntityResourceReleaser  InputPortMessageModes=m  OutputPortMessageModes=m  ResourceToRelease=Selected  ResourceName=Token1
  Scope{1..3,5,7..8,16,21,29,33} (10 alike) : Scope
  Simulink Function1 : Subsystem  TreatAsAtomicUnit=on
  Simulink Function3 : Subsystem  TreatAsAtomicUnit=on
  Stack_Copy : EntityQueue  InputPortMessageModes=m  OutputPortMessageModes=n,m  Capacity=inf  QueueType=LIFO  NumberEntitiesInBlock=on
      settings: OutputPortMap=o1,o5
  Step : EntityServer  InputPortMessageModes=m  OutputPortMessageModes=m  Capacity=1  ServiceTimeValue=0.001  ServiceTimeAttributeName=CommDelay  EntryAction=|  ExitAction=Entity_out(1);  SortingAttributeName=ID
      | Entity_in(1);
      | %gettime(entity.Time);
  Switch : EntityInputSwitch  InputPortMessageModes=m,m,m  OutputPortMessageModes=m  ActivePortSelection=Switch  SwitchingCriterion=From control port
      settings: InputPortMap=u0,u1,u2
  Switch_Logic : Stateflow chart  TreatAsAtomicUnit=on
  Out : Outport
  wires:
  Stack_Copy/2 -> Copy Takt/1(In)
  Simulink Function3/1(ctrl) -> Switch_Logic/1(Entity_in), Scope2/1
  Simulink Function1/1(ctrl) -> Buffer_out/1
  Stack_Copy/1 -> Scope21/1
  Entity Terminator12/1 -> Scope16/1
  Entity Replicator/2 -> Switch/2
  Logic Takt/1(Out) -> Switch_Logic/2(Entity_out), Scope5/1
  Buffer_Copy/2 -> Entity Replicator12/1
  Buffer_out/2 -> Logic Takt/1(In)
  [blocked_entity] -> Path Combiner/2
  Buffer_Gateway/1 -> Scope7/1
  Buffer_out/1 -> Scope33/1
  Entity Replicator/3 -> Entity Terminator12/1
  Switch/1 -> Buffer_Copy/1
  Processing_Delay/1 -> Step/1
  Path Combiner/1 -> Stack_Copy/1
  Entity Replicator/1 -> Measurement/1(measure)
  Measurement/1(Out) -> Out/1
  Entity Replicator12/1 -> Buffer_Gateway/1
  Blocked Entities/1 -> Switch/3
  Buffer_Gateway/2 -> Fast Takt/1(In)
  Entity Terminator1/1 -> Scope3/1
  Blocked Entities/2 -> Entity Replicator10/1
  [new_entity] -> Path Combiner/1
  Entity Replicator10/2 -> [blocked_entity]
  Entity Replicator10/1 -> Entity Terminator/1
  Entity Replicator12/2 -> [new_entity]
  Copy Takt/1(Out) -> Blocked Entities/1
  Buffer_Copy/1 -> Scope8/1
  Entity Terminator/1 -> Scope29/1
  Switch_Logic/1(path) -> [path]
  Step/1 -> Resource Releaser/1
  Resource Acquirer/1 -> Scope1/1
  Fast Takt/1(Out) -> Entity Terminator1/1
  Resource Acquirer/2 -> Processing_Delay/1
  Resource Releaser/1 -> Entity Replicator/1
  In/1 -> Resource Acquirer/1
  [path] -> Switch/1
